simulink model "updateCase"  (R2024b)
settings: Solver=VariableStepAuto  StartTime=0.0  StopTime=10.0  RelTol=1e-3
settings Model: Creator=ryandavis  LastModifiedBy=ryandavis

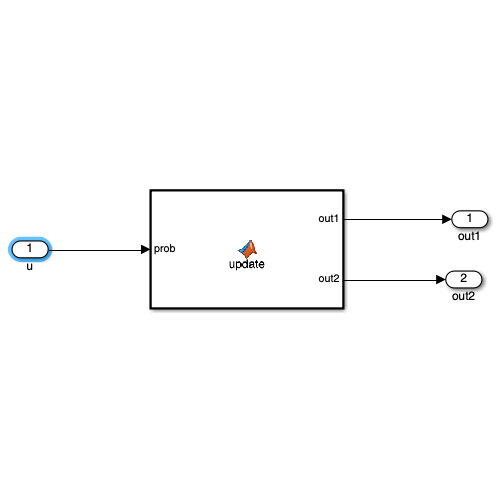
[thumbnail: Simulink's stored preview of the top-level diagram]
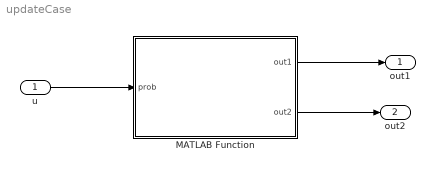
== system updateCase ==
  u : Inport
  MATLAB Function : MATLAB Function  TreatAsAtomicUnit=on
  out1 : Outport
  out2 : Outport  Port=2
  wires:
  u/1 -> MATLAB Function/1(prob)
  MATLAB Function/1(out1) -> out1/1
  MATLAB Function/2(out2) -> out2/1

== matlab function updateCase/MATLAB Function ==
  data: prob input; out1 output; out2 output
function [out1, out2] = update(prob)
    r = rand();
    
    if r < 0.7
        out1 = 1;
        out2 = 0;
    else
        out1 = 0;
        out2 = 1;
    end
end
